simulink model "8_SCR_commutation"  (R2014a)
settings: Solver=ode23tb  StartTime=0.0  StopTime=0.01  RelTol=1e-6
libraries: powerlib x14
settings Model: Creator=CHANDRA BABU  LastModifiedBy=Divya M
settings SolverCC: ZeroCrossControl=DisableAll
settings DataIOCC: SignalLoggingSaveFormat=ModelDataLogs
settings OptimizationCC: ExpressionDepthLimit=2147483647
settings DebuggingCC: UnderspecifiedInitializationDetection=Classic  FcnCallInpInsideContextMsg=UseLocalSettings  StateNameClashWarn=warning
settings GRTTargetCC: CombineOutputUpdateFcns=off  GRTInterface=on

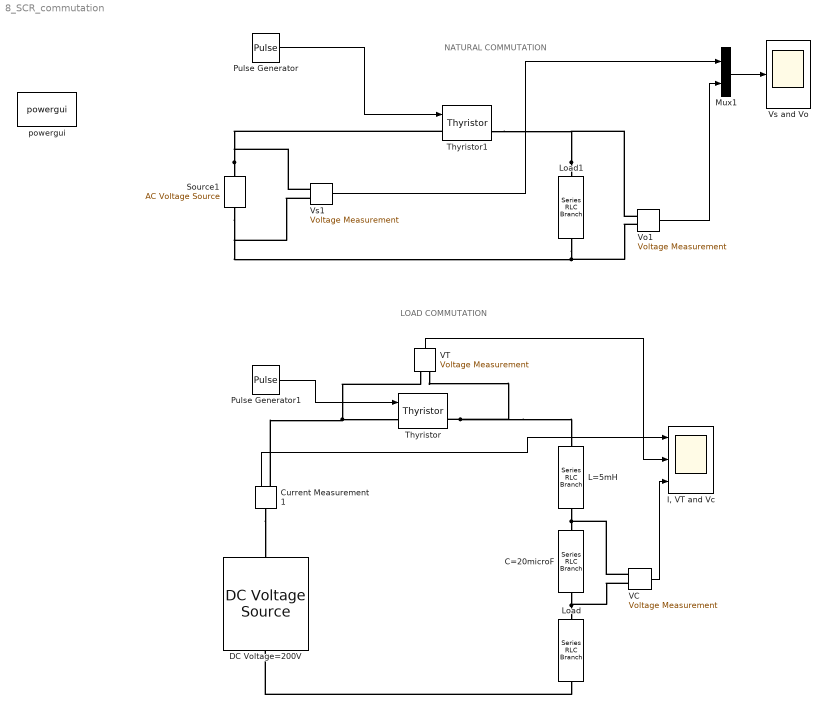
== system 8_SCR_commutation ==
  note: LOAD COMMUTATION
  note: NATURAL COMMUTATION
  " Source1" : powerlib/Electrical Sources/AC Voltage Source  Amplitude=200  Phase=0  Frequency=50  SampleTime=0  Measurements=None
  C=20microF : powerlib/Elements/Series RLC Branch  LConnTagsString=__new0  RConnTagsString=__new0  BranchType=C  Resistance=20  Inductance=5e-3  SetiL0=off  InitialCurrent=0  Capacitance=20e-6  Setx0=off  InitialVoltage=0  Measurements=None
  Current Measurement1 : powerlib/Measurements/Current Measurement  PhasorSimulation=off  OutputType=Complex  PSBequivalent=0
  DC Voltage=200V : powerlib/Electrical Sources/DC Voltage Source  Amplitude=200  Measurements=None
  "I, VT and Vc" : Scope  NumInputPorts=3
      settings: YMin=-5~-250~-5  YMax=15~250~450  SaveName=Outputvoltage
  L=5mH : powerlib/Elements/Series RLC Branch  LConnTagsString=__new0  RConnTagsString=__new0  BranchType=L  Resistance=20  Inductance=5e-3  SetiL0=off  InitialCurrent=0  Capacitance=20e-6  Setx0=off  InitialVoltage=0  Measurements=None
  Load : powerlib/Elements/Series RLC Branch  LConnTagsString=__new0  RConnTagsString=__new0  BranchType=R  Resistance=0.0001  Inductance=5e-3  SetiL0=off  InitialCurrent=0  Capacitance=20e-6  Setx0=off  InitialVoltage=0  Measurements=None
  Load1 : powerlib/Elements/Series RLC Branch  LConnTagsString=__new0  RConnTagsString=__new0  BranchType=R  Resistance=2.5  Inductance=1e-3  SetiL0=off  InitialCurrent=0  Capacitance=1e-6  Setx0=off  InitialVoltage=0  Measurements=None
  Mux1 : Mux  Inputs=2
  Pulse Generator : DiscretePulseGenerator  PulseType=Time based  Period=0.02  PulseWidth=5  PhaseDelay=0.005
  Pulse Generator1 : DiscretePulseGenerator  PulseType=Time based  Period=100e-3  PulseWidth=5  PhaseDelay=0.005
  Thyristor : powerlib/Power Electronics/Thyristor  Ron=0.001  Lon=0  Vf=0.8  IC=0  Rs=500  Cs=250e-9  Measurements=on
  Thyristor1 : powerlib/Power Electronics/Thyristor  Ron=0.001  Lon=0  Vf=0.8  IC=0  Rs=500  Cs=250e-9  Measurements=on
  VC : powerlib/Measurements/Voltage Measurement  PhasorSimulation=off  OutputType=Complex  PSBequivalent=0
  VT : powerlib/Measurements/Voltage Measurement  PhasorSimulation=off  OutputType=Complex  PSBequivalent=0
  Vo1 : powerlib/Measurements/Voltage Measurement  PhasorSimulation=off  OutputType=Complex  PSBequivalent=0
  Vs and Vo : Scope
      settings: SaveName=Outputvoltage1
  Vs1 : powerlib/Measurements/Voltage Measurement  PhasorSimulation=off  OutputType=Complex  PSBequivalent=0
  powergui : powerlib/powergui  Priority=1  SimulationMode=Continuous  SolverType=Tustin  SampleTime=50e-6  frequency=60  SPID=off  DisableSnubberDevices=off  DisableRonSwitches=off  DisableVfSwitches=off  SwTol=0  Interpol=off  DisplayEquations=off  Ts=0  methode=off  frequencyindice=0  Pbase=100e6  ErrMax=1e-4  Iterations=50  UnitsV=kV  UnitsW=MW  FunctionMessages=off  echomessages=off  HookPort=off  EnableUseOfTLC=off  x0status=blocks  RestoreLinks=warning  ResistiveCurrentMeasurement=off  Frange=[0:2:500]  Ylog=off  Xlog=on  ShowGrid=off  save=off  variable=ZData  structure=Outputvoltage  ZoomFFT=on  StartTime=0.0  cycles=1  DisplayStyle=1  fundamental=50  FreqAxis=on  MaxFrequency=1000  frequencyindicesteady=1  RmsSteady=1  display=off
  wires:
  Pulse Generator/1 -> Thyristor1/1
  Vs1/1 -> Mux1/1
  Vo1/1 -> Mux1/2
  Mux1/1 -> Vs and Vo/1
  Pulse Generator1/1 -> Thyristor/1
  VT/1 -> "I, VT and Vc"/2
  VC/1 -> "I, VT and Vc"/3
  Current Measurement1/1 -> "I, VT and Vc"/1
  connections:
  " Source1"/RConn1 -- Thyristor1/LConn1 -- Vs1/LConn1
  Load1/LConn1 -- Thyristor1/RConn1 -- Vo1/LConn1
  Load1/RConn1 -- Vo1/LConn2 -- Vs1/LConn2 -- " Source1"/LConn1
  VT/LConn1 -- Current Measurement1/RConn1 -- Thyristor/LConn1
  Load/RConn1 -- DC Voltage=200V/LConn1
  Thyristor/RConn1 -- VT/LConn2 -- L=5mH/LConn1
  L=5mH/RConn1 -- C=20microF/LConn1 -- VC/LConn1
  C=20microF/RConn1 -- Load/LConn1 -- VC/LConn2
  Current Measurement1/LConn1 -- DC Voltage=200V/RConn1
